simulink model "M182_Lab3"  (R2019b)
settings: Solver=VariableStepAuto  StartTime=0.0  StopTime=1000  RelTol=1e-3
settings Model: Creator=scjcb  LastModifiedBy=scjcb

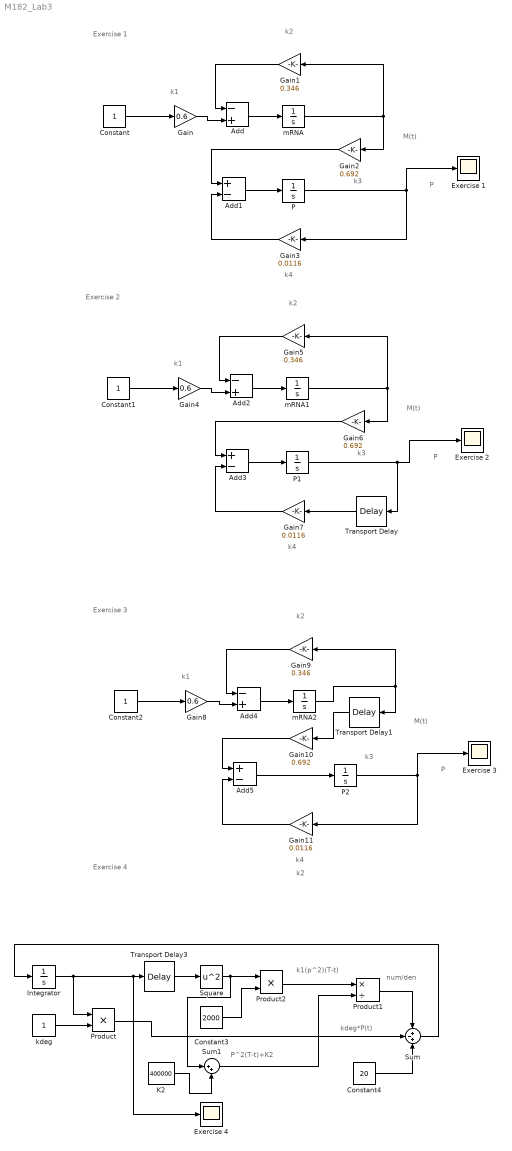
== system M182_Lab3 ==
  note: kdeg*P(t)
  note: num/den
  note: P^2(T-t)+K2
  note: k1(p^2)(T-t)
  note: Exercise 2
  note: Exercise 1
  note: k3
  note: k4
  note: k2
  note: k1
  note: P
  note: M(t)
  note: P
  note: k2
  note: k4
  note: k3
  note: k1
  note: M(t)
  note: Exercise 3
  note: M(t)
  note: k3
  note: k1
  note: k4
  note: P
  note: k2
  note: Exercise 4
  note: k2
  Add : Sum  Inputs=-+
  Add1 : Sum  Inputs=+-
  Add2 : Sum  Inputs=-+
  Add3 : Sum  Inputs=+-
  Add4 : Sum  Inputs=-+
  Add5 : Sum  Inputs=+-
  Constant : Constant
  Constant1 : Constant
  Constant2 : Constant
  Constant3 : Constant  Value=2000
  Constant4 : Constant  Value=20
  Exercise {1..4} (4 alike) : Scope
  Gain : Gain  Gain=0.6
  Gain1 : Gain  Gain=0.346
  Gain10 : Gain  Gain=0.692
  Gain11 : Gain  Gain=0.0116
  Gain2 : Gain  Gain=0.692
  Gain3 : Gain  Gain=0.0116
  Gain4 : Gain  Gain=0.6
  Gain5 : Gain  Gain=0.346
  Gain6 : Gain  Gain=0.692
  Gain7 : Gain  Gain=0.0116
  Gain8 : Gain  Gain=0.6
  Gain9 : Gain  Gain=0.346
  Integrator : Integrator  InitialCondition=200
  "K2 " : Constant  Value=400000
  P : Integrator
  P1 : Integrator
  P2 : Integrator
  Product : Product  Inputs=**
  Product1 : Product  Inputs=*/
  Product2 : Product  Inputs=**
  Square : Math  Operator=square  SignedPower=off  SaturateOnIntegerOverflow=on
  Sum : Sum  Inputs=+-+
  Sum1 : Sum  Inputs=|++
  Transport Delay : TransportDelay  DelayTime=[0,20,40,60,80,100]
  Transport Delay1 : TransportDelay  DelayTime=[0,20,40,60,80,100]
  Transport Delay3 : TransportDelay  DelayTime=[0,5,10,15]  InitialOutput=200
  kdeg : Constant
  mRNA : Integrator
  mRNA1 : Integrator
  mRNA2 : Integrator
  wires:
  Constant/1 -> Gain/1
  Gain/1 -> Add/2
  Add/1 -> mRNA/1
  mRNA/1 -> Gain1/1, Gain2/1
  Gain1/1 -> Add/1
  Gain2/1 -> Add1/1
  Gain3/1 -> Add1/2
  Add1/1 -> P/1
  P/1 -> Exercise 1/1, Gain3/1
  Gain4/1 -> Add2/2
  Add2/1 -> mRNA1/1
  Constant1/1 -> Gain4/1
  P1/1 -> Transport Delay/1, Exercise 2/1
  Gain7/1 -> Add3/2
  mRNA1/1 -> Gain5/1, Gain6/1
  Add3/1 -> P1/1
  Gain5/1 -> Add2/1
  Gain6/1 -> Add3/1
  Transport Delay/1 -> Gain7/1
  P2/1 -> Gain11/1, Exercise 3/1
  Constant2/1 -> Gain8/1
  Add4/1 -> mRNA2/1
  Gain8/1 -> Add4/2
  Gain10/1 -> Add5/1
  Gain11/1 -> Add5/2
  Gain9/1 -> Add4/1
  Add5/1 -> P2/1
  mRNA2/1 -> Transport Delay1/1, Gain9/1
  Transport Delay1/1 -> Gain10/1
  kdeg/1 -> Product/2
  Integrator/1 -> Exercise 4/1, Transport Delay3/1, Product/1
  Transport Delay3/1 -> Square/1
  Square/1 -> Sum1/1, Product2/1
  Constant3/1 -> Product2/2
  Product2/1 -> Product1/1
  Product1/1 -> Sum/1
  Constant4/1 -> Sum/3
  "K2 "/1 -> Sum1/2
  Sum1/1 -> Product1/2
  Product/1 -> Sum/2
  Sum/1 -> Integrator/1
